simulink model "ASMC_sim_CSEI_FTESO"  (R2022a)
settings: Solver=ode4  StartTime=0.0  StopTime=T_final  FixedStep=Ts  RelTol=1e-3
values from neighbouring files (symbols this model uses):
  ASMC_enabled = 1    [ASMC_ESO_sim_CSEI_Scripts.m]    (also in ASMC_FTESO_sim_CSEI_Scripts.m)
  BL = [20 10 10]    [ASMC_ESO_sim_CSEI_Scripts.m]    (also in ASMC_FTESO_sim_CSEI_Scripts.m; SMC_ESO_sim_CSEI_Scripts.m; SMC_sim_CSEI_Scripts.m)
  Control_allocation = 1    [ASMC_ESO_sim_CSEI_Scripts.m]    (also in ASMC_FTESO_sim_CSEI_Scripts.m; SMC_ESO_sim_CSEI_Scripts.m; SMC_sim_CSEI_Scripts.m)
  current = [0;0]    [ASMC_ESO_sim_CSEI_Scripts.m]    (also in ASMC_FTESO_sim_CSEI_Scripts.m; Berthing_Control_PID_CSEI_Scripts.m; Position_Control_PID_CSEI_Scripts.m; Position_Control_PID_CSEI_Scripts_released.m)
  Disturbance_enabled = 1    [ASMC_ESO_sim_CSEI_Scripts.m]    (also in ASMC_FTESO_sim_CSEI_Scripts.m; SMC_ESO_sim_CSEI_Scripts.m)
  disturbance_type = 0    [ASMC_ESO_sim_CSEI_Scripts.m]    (also in ASMC_FTESO_sim_CSEI_Scripts.m = 2)
  ESO_enabled = 1    [ASMC_ESO_sim_CSEI_Scripts.m]    (also in ASMC_FTESO_sim_CSEI_Scripts.m; SMC_ESO_sim_CSEI_Scripts.m = 0)
  ESO_type = 2    [ASMC_FTESO_sim_CSEI_Scripts.m]
  ESO_type_enabled = 1    [ASMC_FTESO_sim_CSEI_Scripts.m]
  k1_init = 0.1*[5;5;10]    [ASMC_ESO_sim_CSEI_Scripts.m]    (also in ASMC_FTESO_sim_CSEI_Scripts.m)
  k2 = [5;5;5]    [ASMC_ESO_sim_CSEI_Scripts.m]    (also in ASMC_FTESO_sim_CSEI_Scripts.m)
  k3 = 0.05*[10; 20; 50]    [ASMC_ESO_sim_CSEI_Scripts.m]    (also in ASMC_FTESO_sim_CSEI_Scripts.m)
  k_min = 1    [ASMC_ESO_sim_CSEI_Scripts.m]    (also in ASMC_FTESO_sim_CSEI_Scripts.m)
  K_SMC = [20 20 50]    [ASMC_ESO_sim_CSEI_Scripts.m]    (also in ASMC_FTESO_sim_CSEI_Scripts.m; SMC_ESO_sim_CSEI_Scripts.m; SMC_sim_CSEI_Scripts.m)
  lamda = [5.0 5.0 10]    [ASMC_ESO_sim_CSEI_Scripts.m]    (also in ASMC_FTESO_sim_CSEI_Scripts.m; SMC_ESO_sim_CSEI_Scripts.m; SMC_sim_CSEI_Scripts.m)
  mu = [0.005; 0.005; 0.005]    [ASMC_ESO_sim_CSEI_Scripts.m]    (also in ASMC_FTESO_sim_CSEI_Scripts.m)
  option = 0    [ASMC_ESO_sim_CSEI_Scripts.m]    (also in ASMC_FTESO_sim_CSEI_Scripts.m; SMC_ESO_sim_CSEI_Scripts.m = 1; SMC_sim_CSEI_Scripts.m = 1)
  psi_ref = 40    [ASMC_ESO_sim_CSEI_Scripts.m]    (also in ASMC_FTESO_sim_CSEI_Scripts.m; SMC_ESO_sim_CSEI_Scripts.m; SMC_sim_CSEI_Scripts.m)
  tau_max = 20*[3; 3; 3]    [ASMC_ESO_sim_CSEI_Scripts.m]    (also in ASMC_FTESO_sim_CSEI_Scripts.m; SMC_ESO_sim_CSEI_Scripts.m; SMC_sim_CSEI_Scripts.m)
  v_max = 10    [ASMC_ESO_sim_CSEI_Scripts.m]    (also in ASMC_FTESO_sim_CSEI_Scripts.m; Position_Control_PID_CSEI_Scripts.m = 2; Position_Control_PID_CSEI_Scripts_released.m = 2; SMC_ESO_sim_CSEI_Scripts.m)
  w0 = 60    [ASMC_ESO_sim_CSEI_Scripts.m]    (also in ASMC_FTESO_sim_CSEI_Scripts.m; SMC_ESO_sim_CSEI_Scripts.m)
  w0_FTESO = 10    [ASMC_FTESO_sim_CSEI_Scripts.m]
  w_d = 0.5    [ASMC_ESO_sim_CSEI_Scripts.m]    (also in ASMC_FTESO_sim_CSEI_Scripts.m; SMC_ESO_sim_CSEI_Scripts.m; SMC_sim_CSEI_Scripts.m)
  x0 = zeros(6,1)    [Berthing_Control_PID_CSEI_Scripts.m]    (also in Position_Control_PID_CSEI_Scripts.m; Position_Control_PID_CSEI_Scripts_released.m; Waypoint_Control_PID_CSEI_Scripts.m; Waypoint_Control_PID_CSEI_Scripts_LLA.m)
  x_ref = 7    [ASMC_ESO_sim_CSEI_Scripts.m]    (also in ASMC_FTESO_sim_CSEI_Scripts.m; SMC_ESO_sim_CSEI_Scripts.m; SMC_sim_CSEI_Scripts.m)
  y_ref = 7    [ASMC_ESO_sim_CSEI_Scripts.m]    (also in ASMC_FTESO_sim_CSEI_Scripts.m; SMC_ESO_sim_CSEI_Scripts.m; SMC_sim_CSEI_Scripts.m)
  zeta_d = 1    [ASMC_ESO_sim_CSEI_Scripts.m]    (also in ASMC_FTESO_sim_CSEI_Scripts.m; SMC_ESO_sim_CSEI_Scripts.m; SMC_sim_CSEI_Scripts.m)
undefined symbols (not defined in the file or in its folder): sigbuilder_block
libraries: simulink_extras x5
(part 2 of 2)

== matlab function ASMC_sim_CSEI_FTESO/control allocation/Force_Moment ==
  data: tau input; u output; alpha output; tau_max input
function [u, alpha] = force2input(tau, tau_max)
    % Mapping of desired force (tau) to input to the actuators (u)
    % Input: 3DOF desired forces and moment in body-frame, tau = [X Y N]'
    % Output: input signals to the actuators, u = [u_BT u_VSP1 u_VSP2]';
    %         angles of the two VSPs, alpha = [alpha_VSP1 alpha_VSP2]';
    %         angular rates of the VSPs, omega = [omega_VSP1 omega_VSP2]'
    %
    % Author: Caroline Fleischer, Elias Gauslaa, Jakob Jensen
    % Date:   20.02.2020

%% Initializing values
    ly_VSP = 0.055;         % Moment arm along y for VSP
    lx_VSP = 0.4574;        % Moment arm along x for VSP
    lx_BT = 0.3875;         % Moment arm along x for BT
    
    % default
%     f_VSP1_max = 0.45;      % Max thrust VSP1 
%     f_VSP2_max = 0.45;      % Max thrust VSP2
%     f_BT_max = 0.3;         % Max thrust BT
%     
    % test
    f_VSP1_max = tau_max(2);      % Max thrust VSP1
    f_VSP2_max = tau_max(3);      % Max thrust VSP2
    f_BT_max = tau_max(1);         % Max thrust BT

%     omega_VSP1 = 0.199;     % Rotation speed for VSP1, LABORATORY ONLY
%     omega_VSP2 = 0.235;     % Rotation speed for VSP2, LABORATORY ONLY
    alpha = zeros(2,1);     % VSP angles
%     omega = zeros(2,1);     % VSP angular rates
    u = zeros(3,1);         % Input vector to the VSPs and BT

    B = [  1      0       1      0      0;
           0      1       0      1      1;
         ly_VSP -lx_VSP -ly_VSP -lx_VSP lx_BT]; % Configuration matrix
%% Thrust allocation
    B_dagger = pinv(B);                         % Calculating dagger

    %f_vps1,x f_vps1,y, 
    f_cmd = B_dagger*tau;                       % Forces and moment

    u_cmd = [norm(f_cmd(1:2))/f_VSP1_max;
             norm(f_cmd(3:4))/f_VSP2_max;
             f_cmd(5)/f_BT_max];                % Calculating input to each
                                                % thruster

    % Saturation: Limit input signal to VSPs to be within [0,1]
    if u_cmd(1) < 0
        u_cmd(1) = 0;
    elseif u_cmd(1) > 1
        u_cmd(1) = 1;
    else
        u_cmd(1) = u_cmd(1);
    end

    if u_cmd(2) < 0
        u_cmd(2) = 0;
    elseif u_cmd(2) > 1
        u_cmd(2) = 1;
    else
        u_cmd(2) = u_cmd(2);
    end

    % Saturation: Limit input signal to BT to be within [-1,1]
    if u_cmd(3) < -1
        u_cmd(3) = -1;
    elseif u_cmd(3) > 1
        u_cmd(3) = 1;
    else
        u_cmd(3) = u_cmd(3);
    end
    
    alpha(1) = atan2(f_cmd(2),f_cmd(1));         % Calculate angle of VSP1
    alpha(2) = atan2(f_cmd(4),f_cmd(3));         % Calculate angle of VSP2
    
%     omega(1) = omega_VSP1;                       % Output omega LAB ONLY
%     omega(2) = omega_VSP2;                       % Output omega LAB ONLY

    BT_gain = 1;                                 % Gain used in LAB

    u(1) = u_cmd(3)*BT_gain;                     % Output input to BT
    u(2) = u_cmd(1);                             % Output input to VSP1
    u(3) = u_cmd(2);                             % Output input to VSP2
    
end

== matlab function ASMC_sim_CSEI_FTESO/ASMC/SMC ==
  data: ME input; tau output; tau_sw output; CE input; DE input; GE input; eta_dot input; eta_ddot input; e input; e_dot input; e_ddot input; lamda input; K_SMC input; BL input; option input; s output; d_hat input
function [tau, tau_sw, s] = SMC(ME, CE, DE, GE, eta_dot, eta_ddot, e, e_dot, e_ddot, lamda, K_SMC, BL, option, d_hat)


%  u:     surge velocity          (m/s)
%  v:     sway velocity           (m/s)
%  w:     heave velocity          (m/s)
%  p:     roll velocity           (rad/s)
%  q:     pitch velocity          (rad/s)
%  r:     yaw velocity            (rad/s)
%  x:     position in x direction (m)
%  y:     position in y direction (m)
%  z:     position in z direction (m)
%  phi:   roll angle              (rad)
%  theta: pitch angle             (rad)
%  psi:   yaw angle               (rad)


s = e_dot + lamda.*e;
s_dot = e_ddot + lamda.*e_dot;

tau_eq = ME*(eta_ddot+s_dot)+(CE+DE)*(eta_dot+s)+GE  - d_hat;

if option == 1
    tau_sw = K_SMC.*tanh(s./BL);
elseif option == 2
    tau_sw = K_SMC.*sign(s);
else 
    tau_sw = [0;0;0];
end


tau = tau_eq + tau_sw;

== matlab function ASMC_sim_CSEI_FTESO/MATLAB Function3 ==
  data: psi input; psi_mod output
function psi_mod = wrapToPi(psi)

psi_mod = mod(psi + pi, 2*pi) - pi;
